simulink library "lib_discrete_time_PI_controller"  (R2023a)
settings: Solver=VariableStepAuto  StartTime=0.0  StopTime=10.0  RelTol=1e-3
undefined symbols (not defined in the file): bit
libraries: lib_conversion x11, lib_dynamic_saturator x4, lib_discrete_time_integrator x4
settings Model: Creator=cav2ofo  LastModifiedBy=xiaoqiang.yuan
settings OptimizationCC: ReuseModelBlockBuffer=off

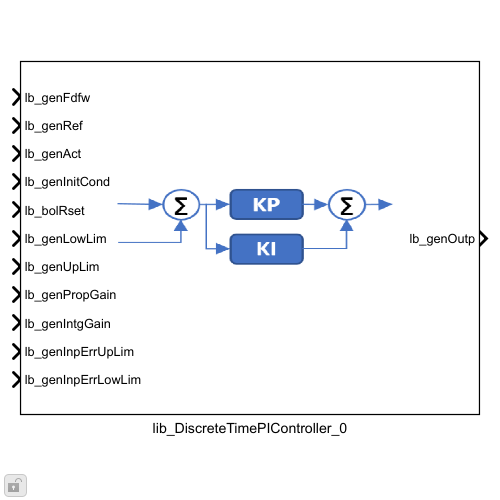
[thumbnail: Simulink's stored preview of the top-level diagram]
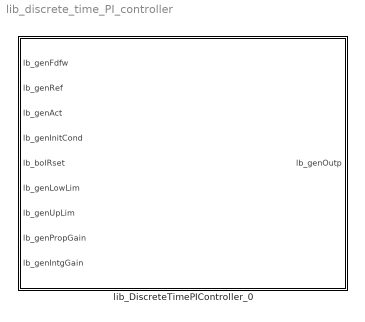
== system lib_discrete_time_PI_controller ==
  lib_DiscreteTimePIController_0 : Subsystem  mask{lb_parSampTime=0.01, lb_parMaxSampTime=0.1, lb_parMaxPropGain=1, lb_parMaxIntgGain=1, lb_parRefInpMaxVal=1000, lb_parRefInpMinVal=-1000, lb_parMaxErrVal=2*1000, lb_parMinErrVal=-2*1000, lb_parMaxOutpVal=20, lb_parMinOutpVal=-20, lb_parAccmDataTypeMode=32-bit, lb_parOutpDataType=fixdt(1,16,2^0,0), lb_parSatMode=anti-windup with back-calculation}
      mask prompts: lb_parSampTime "Sampling time [s]:"; lb_parMaxSampTime "Maximum sampling time [s]:"; lb_parMaxPropGain "Maximum proportional gain (kp):"; lb_parMaxIntgGain "Maximum integral gain [ou/(iu*s)]:"; lb_parRefInpMaxVal "Reference input maximum value [iu]:"; lb_parRefInpMinVal "Reference input minimum value [iu]:"; lb_parMaxErrVal "Maximum error (Ref-Act) value [iu]:"; lb_parMinErrVal "Minimum error (Ref-Act) value [iu]:"; lb_parMaxOutpVal "Maximum output value [ou]:"; lb_parMinOutpVal "Minimum output value [ou]:"; lb_parAccmDataTypeMode "Accumulator data type mode:"; lb_parOutpDataType "Output data type:"; lb_parSatMode "Output saturation mode:"
      mask init:
      | % =======================================================
      | % This script is a script to flags output saturation
      | % when either the output saturation without anti-windup
      | % or custom anti-windup method is selected. It also computes
      | % custom datatypes required for intermediate calcuations
      | % Author: Niraj Rathod
      | % Date: 19/07/2022
      | % =======================================================
      | % Enable saturation flag in case of saturation 
      | % without anti-windup (2) or custom anti-windup method (4)
      | % if lb_parAntiWdpMtd == 2 ||  lb_parAntiWdpMtd == 4
      | %    set_param(gcb,'lb_parSatFlag', 'on');
      | % else
      | %    set_param(gcb,'lb_parSatFlag', 'off');
      | % end
      | 
      | % Setting the maximum sampling time equal to the user define sampling time
      | % value
      | lb_parMaxSampTime = double(lb_parSampTime);
      | 
      | % Data type slope for the diffference between unstaurated 
      | % and saturated output signal used by anti-windup 
      | % with back-calculation
      | lb_outpDiffDataType = Simulink.NumericType;
      | lb_outpDiffDataType.DataTypeMode = 'Fixed-point: slope and bias scaling';
      | lb_outpDiffDataType.Slope = lb_parOutpDataType.Slope*2; 
      | 
      | % Min/max value for accumulator datatype
      | lb_parAccmMaxOutp = 3*double(lb_parRefInpMaxVal);
      | lb_parAccmMinOutp = 3*double(lb_parRefInpMinVal);
      | 
      | 
      | %% Activate variant subsystem choice by means of set_param function
      | % switch lb_parSatMode
      | %     
      | %     case 'none' 
      | %         
      | %         set_param([gcb,'/vss_PIControllerModes'],'VariantControl', 'VSS_MODE == 1')
      | %         set_param(gcb,'lb_parSatFlag', 'off');
      | % 
      | %     case 'output saturation without anti-windup'
      | % 
      | %         set_param([gcb,'/vss_PIControllerModes'],'VariantControl', 'VSS_MODE == 1')
      | %         set_param(gcb,'lb_parSatFlag', 'on');
      | % 
      | %     case 'anti-windup with custom algorithm'
      | %         
      | %         set_param([gcb,'/vss_PIControllerModes'],'VariantControl', 'VSS_MODE == 2')
      | %         set_param(gcb,'lb_parSatFlag', 'off');
      | %         
      | %     case 'Integral control'
      | %         
      | %         set_param([gcb,'/vss_PIControllerModes'],'VariantControl', 'VSS_MODE == 3')
      | %         set_param(gcb,'lb_parSatFlag', 'off');
      | %         
      | % end
      mask TypeOptions lb_parMaxSampTime: vss_PIControllerModes/vss_NoSaturation/lib_DiscreteTimeIntegrator_1/lb_parMaxSampTime | vss_PIControllerModes/vss_SaturationBackCalcAntiWindup/lib_DiscreteTimeIntegrator_1/lb_parMaxSampTime | vss_PIControllerModes/vss_SaturationCustomAntiWindup/lib_DiscreteTimeIntegrator_1/lb_parMaxSampTime | vss_PIControllerModes/vss_SaturationNoAntiWindup/lib_DiscreteTimeIntegrator_1/lb_parMaxSampTime
      mask TypeOptions lb_parMaxIntgGain: vss_PIControllerModes/vss_NoSaturation/lib_DiscreteTimeIntegrator_1/lb_parMaxIntgGain | vss_PIControllerModes/vss_SaturationBackCalcAntiWindup/lib_DiscreteTimeIntegrator_1/lb_parMaxIntgGain | vss_PIControllerModes/vss_SaturationCustomAntiWindup/lib_DiscreteTimeIntegrator_1/lb_parMaxIntgGain | vss_PIControllerModes/vss_SaturationNoAntiWindup/lib_DiscreteTimeIntegrator_1/lb_parMaxIntgGain
      mask TypeOptions lb_parAccmDataTypeMode: vss_PIControllerModes/vss_NoSaturation/lib_DiscreteTimeIntegrator_1/lb_parAccmDataTypeMode | vss_PIControllerModes/vss_SaturationBackCalcAntiWindup/lib_DiscreteTimeIntegrator_1/lb_parAccmDataTypeMode | vss_PIControllerModes/vss_SaturationCustomAntiWindup/lib_DiscreteTimeIntegrator_1/lb_parAccmDataTypeMode | vss_PIControllerModes/vss_SaturationNoAntiWindup/lib_DiscreteTimeIntegrator_1/lb_parAccmDataTypeMode
      mask TypeOptions lb_parSatMode: none | output saturation without anti-windup | anti-windup with back-calculation | anti-windup with custom algorithm
      mask DialogControl DescGroupVar Prompt: Proportional-Integral (PI) Controller
      mask DialogControl DescTextVar Prompt: VHIT Control Library
      mask DialogControl piDesc Prompt: This is a Custom Proportional-Integral (PI) block developed for the motor control.
      mask DialogControl blockParam Prompt: Parameters
      mask DialogControl dataTypeDesc Prompt: Data type
      mask DialogControl oprModDesc Prompt: Operating modes
      mask Display: image('PiController.png')

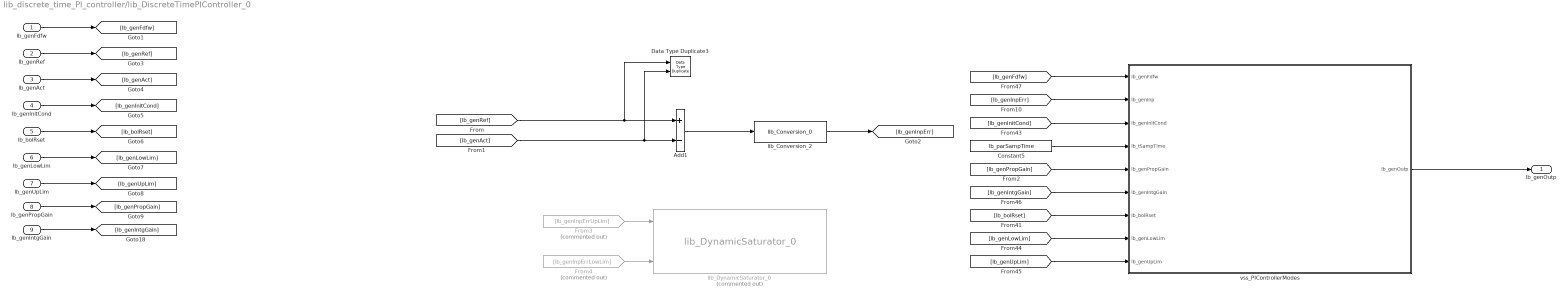
== system lib_discrete_time_PI_controller/lib_DiscreteTimePIController_0 ==
  lb_genFdfw : Inport  OutDataTypeStr=lb_parOutpDataType
  lb_genRef : Inport  Port=2  OutMin=lb_parRefInpMinVal  OutMax=lb_parRefInpMaxVal
  lb_genAct : Inport  Port=3  OutMin=lb_parRefInpMinVal  OutMax=lb_parRefInpMaxVal
  lb_genInitCond : Inport  Port=4  OutDataTypeStr=lb_parOutpDataType
  lb_bolRset : Inport  Port=5  OutDataTypeStr=boolean
  lb_genLowLim : Inport  Port=6  OutDataTypeStr=lb_parOutpDataType
  lb_genUpLim : Inport  Port=7  OutDataTypeStr=lb_parOutpDataType
  lb_genPropGain : Inport  Port=8  OutMin=0  OutMax=lb_parMaxPropGain
  lb_genIntgGain : Inport  Port=9  OutMin=0  OutMax=lb_parMaxIntgGain
  Add1 : Sum  Inputs=+-  OutDataTypeStr=Inherit: Inherit via back propagation  RndMeth=Simplest
  Constant5 : Constant  Value=lb_parSampTime
  Data Type Duplicate3 : DataTypeDuplicate
  From3 : From  Commented=on  GotoTag=lb_genInpErrUpLim
  From4 : From  Commented=on  GotoTag=lb_genInpErrLowLim
  lib_Conversion_2 : lib_conversion/lib_Conversion_0  lb_parDataType=fixdt(1,16)  lb_parOutpMaxVal=2*lb_parRefInpMaxVal  lb_parOutpMinVal=2*lb_parRefInpMinVal  lb_parSatFlag=off
  lib_DynamicSaturator_0 : lib_dynamic_saturator/lib_DynamicSaturator_0  Commented=on
  vss_PIControllerModes : Subsystem  Variant=on
  lb_genOutp : Outport  VectorParamsAs1DForOutWhenUnconnected=off
  wires:
  [lb_genPropGain] -> vss_PIControllerModes/5(lb_genPropGain)
  lb_genPropGain/1 -> [lb_genPropGain]
  lb_genLowLim/1 -> [lb_genLowLim]
  lb_genUpLim/1 -> [lb_genUpLim]
  [lb_genAct] -> Data Type Duplicate3/2, Add1/2
  [lb_genRef] -> Add1/1, Data Type Duplicate3/1
  lb_genRef/1 -> [lb_genRef]
  lb_genAct/1 -> [lb_genAct]
  lb_genInitCond/1 -> [lb_genInitCond]
  lb_bolRset/1 -> [lb_bolRset]
  lb_genFdfw/1 -> [lb_genFdfw]
  lb_genIntgGain/1 -> [lb_genIntgGain]
  [lb_genInpErr] -> vss_PIControllerModes/2(lb_genInp)
  [lb_genInitCond] -> vss_PIControllerModes/3(lb_genInitCond)
  Constant5/1 -> vss_PIControllerModes/4(lb_tSampTime)
  [lb_genIntgGain] -> vss_PIControllerModes/6(lb_genIntgGain)
  [lb_bolRset] -> vss_PIControllerModes/7(lb_bolRset)
  [lb_genLowLim] -> vss_PIControllerModes/8(lb_genLowLim)
  [lb_genUpLim] -> vss_PIControllerModes/9(lb_genUpLim)
  [lb_genFdfw] -> vss_PIControllerModes/1(lb_genFdfw)
  vss_PIControllerModes/1(lb_genOutp) -> lb_genOutp/1
  From3/1 -> lib_DynamicSaturator_0/1
  From4/1 -> lib_DynamicSaturator_0/3
  lib_Conversion_2/1 -> [lb_genInpErr]
  Add1/1 -> lib_Conversion_2/1

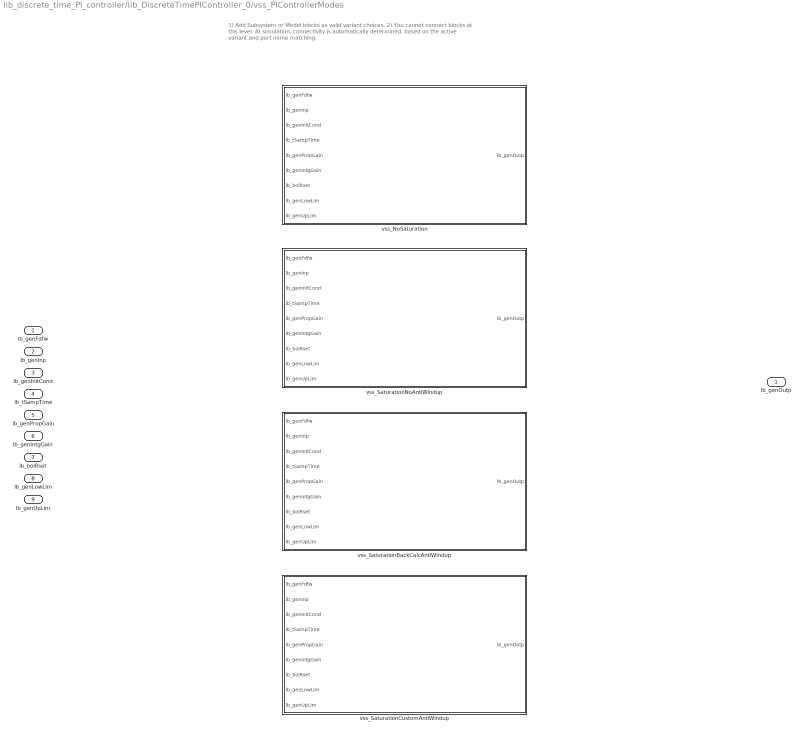
== system lib_discrete_time_PI_controller/lib_DiscreteTimePIController_0/vss_PIControllerModes ==
  note: 1) Add Subsystem or Model blocks as valid variant choices.
      | 2) You cannot connect blocks at this level. At simulation, connectivity is automatically
      | determined, based on the active variant and port name matching.
  lb_genFdfw : Inport
  lb_genInp : Inport  Port=2
  lb_genInitCond : Inport  Port=3
  lb_tSampTime : Inport  Port=4
  lb_genPropGain : Inport  Port=5
  lb_genIntgGain : Inport  Port=6
  lb_bolRset : Inport  Port=7
  lb_genLowLim : Inport  Port=8
  lb_genUpLim : Inport  Port=9
  vss_NoSaturation : Subsystem  VariantControl=lb_parSatMode == 1
  vss_SaturationBackCalcAntiWindup : Subsystem  VariantControl=lb_parSatMode == 3
  vss_SaturationCustomAntiWindup : Subsystem  VariantControl=lb_parSatMode == 4
  vss_SaturationNoAntiWindup : Subsystem  VariantControl=lb_parSatMode == 2
  lb_genOutp : Outport

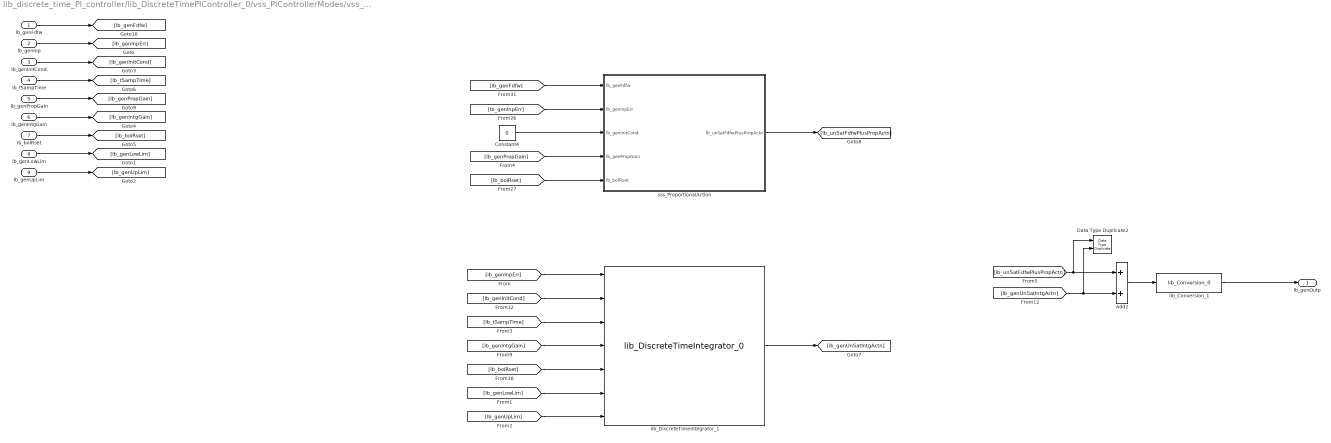
== system lib_discrete_time_PI_controller/lib_DiscreteTimePIController_0/vss_PIControllerModes/vss_NoSaturation ==
  lb_genFdfw : Inport
  lb_genInp : Inport  Port=2
  lb_genInitCond : Inport  Port=3
  lb_tSampTime : Inport  Port=4
  lb_genPropGain : Inport  Port=5
  lb_genIntgGain : Inport  Port=6
  lb_bolRset : Inport  Port=7
  lb_genLowLim : Inport  Port=8
  lb_genUpLim : Inport  Port=9
  Add2 : Sum  OutDataTypeStr=Inherit: Inherit via back propagation  RndMeth=Simplest
  Constant4 : Constant  Value=0  OutDataTypeStr=lb_parOutpDataType
  Data Type Duplicate2 : DataTypeDuplicate
  lib_Conversion_1 : lib_conversion/lib_Conversion_0  lb_parDataType=lb_parOutpDataType  lb_parOutpMaxVal=[]  lb_parOutpMinVal=[]  lb_parSatFlag=off
  lib_DiscreteTimeIntegrator_1 : lib_discrete_time_integrator/lib_DiscreteTimeIntegrator_0  lb_parMaxInpVal=lb_parMaxErrVal  lb_parMinInpVal=lb_parMinErrVal  lb_parMaxSampTime=lb_parMaxSampTime  lb_parMaxIntgGain=lb_parMaxIntgGain  lb_parAccmDataTypeMode=32-bit  lb_parOutpDataType=lb_parOutpDataType  lb_parIntgScopMode=Integral control  lb_parSatFlag=off
      settings: LibrarySourceBlock=vhit_control_library/lib_DiscreteTimeIntegrator_0
  sss_ProportionalAction : Subsystem
  lb_genOutp : Outport  VectorParamsAs1DForOutWhenUnconnected=off
  wires:
  [lb_genPropGain] -> sss_ProportionalAction/4(lb_genPropGain)
  lb_genPropGain/1 -> [lb_genPropGain]
  [lb_bolRset] -> lib_DiscreteTimeIntegrator_1/5
  [lb_genInpErr] -> lib_DiscreteTimeIntegrator_1/1
  [lb_genLowLim] -> lib_DiscreteTimeIntegrator_1/6
  [lb_genInitCond] -> lib_DiscreteTimeIntegrator_1/2
  [lb_genIntgGain] -> lib_DiscreteTimeIntegrator_1/4
  [lb_tSampTime] -> lib_DiscreteTimeIntegrator_1/3
  lib_DiscreteTimeIntegrator_1/1 -> [lb_genUnSatIntgActn]
  [lb_genUpLim] -> lib_DiscreteTimeIntegrator_1/7
  [lb_genInpErr] -> sss_ProportionalAction/2(lb_genInpErr)
  [lb_bolRset] -> sss_ProportionalAction/5(lb_bolRset)
  [lb_genFdfw] -> sss_ProportionalAction/1(lb_genFdfw)
  sss_ProportionalAction/1(lb_unSatFdfwPlusPropActn) -> [lb_unSatFdfwPlusPropActn]
  Constant4/1 -> sss_ProportionalAction/3(lb_genInitCond)
  Add2/1 -> lib_Conversion_1/1
  [lb_unSatFdfwPlusPropActn] -> Data Type Duplicate2/1, Add2/1
  [lb_genUnSatIntgActn] -> Add2/2, Data Type Duplicate2/2
  lib_Conversion_1/1 -> lb_genOutp/1
  lb_genInp/1 -> [lb_genInpErr]
  lb_genInitCond/1 -> [lb_genInitCond]
  lb_tSampTime/1 -> [lb_tSampTime]
  lb_genIntgGain/1 -> [lb_genIntgGain]
  lb_bolRset/1 -> [lb_bolRset]
  lb_genLowLim/1 -> [lb_genLowLim]
  lb_genUpLim/1 -> [lb_genUpLim]
  lb_genFdfw/1 -> [lb_genFdfw]

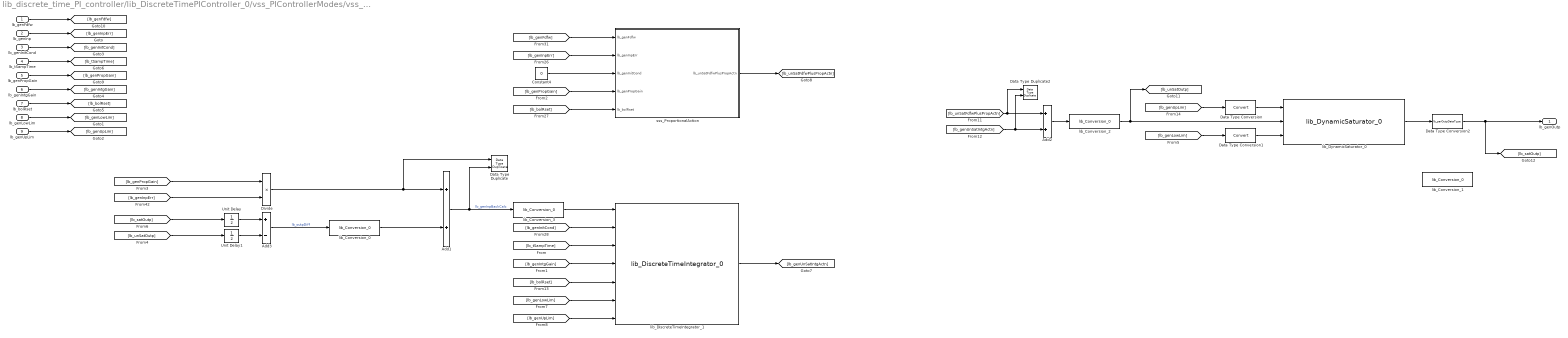
== system lib_discrete_time_PI_controller/lib_DiscreteTimePIController_0/vss_PIControllerModes/vss_SaturationBackCalcAntiWindup ==
  lb_genFdfw : Inport
  lb_genInp : Inport  Port=2
  lb_genInitCond : Inport  Port=3
  lb_tSampTime : Inport  Port=4
  lb_genPropGain : Inport  Port=5
  lb_genIntgGain : Inport  Port=6
  lb_bolRset : Inport  Port=7
  lb_genLowLim : Inport  Port=8
  lb_genUpLim : Inport  Port=9
  Add1 : Sum  OutDataTypeStr=Inherit: Inherit via back propagation  RndMeth=Simplest
  Add2 : Sum  OutDataTypeStr=Inherit: Inherit via back propagation  RndMeth=Simplest
  Add3 : Sum  Inputs=+-  OutDataTypeStr=Inherit: Inherit via back propagation  RndMeth=Simplest
  Constant4 : Constant  Value=0  OutDataTypeStr=Inherit: Inherit via back propagation
  Data Type Duplicate : DataTypeDuplicate
  Data Type Duplicate2 : DataTypeDuplicate
  Data Type Conversion : DataTypeConversion  SaturateOnIntegerOverflow=off  RndMeth=Floor
  Data Type Conversion1 : DataTypeConversion  SaturateOnIntegerOverflow=off  RndMeth=Floor
  Data Type Conversion2 : DataTypeConversion  OutDataTypeStr=lb_parOutpDataType  SaturateOnIntegerOverflow=off  RndMeth=Floor
  Divide : Product  Inputs=**  OutDataTypeStr=Inherit: Inherit via back propagation
  Unit Delay : UnitDelay  SampleTime=-1  HasFrameUpgradeWarning=on
  Unit Delay1 : UnitDelay  SampleTime=-1  HasFrameUpgradeWarning=on
  lib_Conversion_0 : lib_conversion/lib_Conversion_0  lb_parDataType=lb_outpDiffDataType  lb_parOutpMaxVal=[]  lb_parOutpMinVal=[]  lb_parSatFlag=off
  lib_Conversion_1 : lib_conversion/lib_Conversion_0  lb_parDataType=lb_parOutpDataType  lb_parOutpMaxVal=[]  lb_parOutpMinVal=[]  lb_parSatFlag=off
  lib_Conversion_2 : lib_conversion/lib_Conversion_0  lb_parDataType=lb_outpDiffDataType  lb_parOutpMaxVal=[]  lb_parOutpMinVal=[]  lb_parSatFlag=off
  lib_Conversion_3 : lib_conversion/lib_Conversion_0  lb_parDataType=lb_parOutpDataType  lb_parOutpMaxVal=[]  lb_parOutpMinVal=[]  lb_parSatFlag=off
  lib_DiscreteTimeIntegrator_1 : lib_discrete_time_integrator/lib_DiscreteTimeIntegrator_0  lb_parMaxInpVal=lb_parMaxOutpVal  lb_parMinInpVal=-lb_parMaxOutpVal  lb_parMaxSampTime=lb_parMaxSampTime  lb_parMaxIntgGain=lb_parMaxIntgGain  lb_parAccmDataTypeMode=32-bit  lb_parOutpDataType=lb_parOutpDataType  lb_parIntgScopMode=Integral control  lb_parSatFlag=off
      settings: LibrarySourceBlock=vhit_control_library/lib_DiscreteTimeIntegrator_0
  lib_DynamicSaturator_0 : lib_dynamic_saturator/lib_DynamicSaturator_0
  sss_ProportionalAction : Subsystem
  lb_genOutp : Outport  VectorParamsAs1DForOutWhenUnconnected=off
  wires:
  [lb_genInpErr] -> sss_ProportionalAction/2(lb_genInpErr)
  Constant4/1 -> sss_ProportionalAction/3(lb_genInitCond)
  sss_ProportionalAction/1(lb_unSatFdfwPlusPropActn) -> [lb_unSatFdfwPlusPropActn]
  [lb_bolRset] -> sss_ProportionalAction/5(lb_bolRset)
  [lb_genFdfw] -> sss_ProportionalAction/1(lb_genFdfw)
  [lb_genPropGain] -> sss_ProportionalAction/4(lb_genPropGain)
  lb_genPropGain/1 -> [lb_genPropGain]
  lb_genIntgGain/1 -> [lb_genIntgGain]
  Data Type Conversion2/1 -> lb_genOutp/1, [lb_satOutp]
  lb_genFdfw/1 -> [lb_genFdfw]
  lb_genUpLim/1 -> [lb_genUpLim]
  lb_genInitCond/1 -> [lb_genInitCond]
  lb_bolRset/1 -> [lb_bolRset]
  lb_genInp/1 -> [lb_genInpErr]
  lb_genLowLim/1 -> [lb_genLowLim]
  lb_tSampTime/1 -> [lb_tSampTime]
  lib_DiscreteTimeIntegrator_1/1 -> [lb_genUnSatIntgActn]
  [lb_tSampTime] -> lib_DiscreteTimeIntegrator_1/3
  [lb_unSatOutp] -> Unit Delay1/1
  Add3/1 -> lib_Conversion_0/1  "lb_outpDiff"
  Add1/1 -> lib_Conversion_3/1, Data Type Duplicate/2  "lb_genInpBackCalc"
  Divide/1 -> Add1/1, Data Type Duplicate/1
  [lb_satOutp] -> Unit Delay/1
  [lb_bolRset] -> lib_DiscreteTimeIntegrator_1/5
  lib_Conversion_3/1 -> lib_DiscreteTimeIntegrator_1/1
  [lb_genInpErr] -> Divide/2
  [lb_genIntgGain] -> lib_DiscreteTimeIntegrator_1/4
  [lb_genInitCond] -> lib_DiscreteTimeIntegrator_1/2
  [lb_genUnSatIntgActn] -> Add2/2, Data Type Duplicate2/2
  lib_DynamicSaturator_0/1 -> Data Type Conversion2/1
  [lb_genLowLim] -> Data Type Conversion1/1
  [lb_genUpLim] -> Data Type Conversion/1
  [lb_unSatFdfwPlusPropActn] -> Data Type Duplicate2/1, Add2/1
  [lb_genLowLim] -> lib_DiscreteTimeIntegrator_1/6
  [lb_genUpLim] -> lib_DiscreteTimeIntegrator_1/7
  Unit Delay/1 -> Add3/1
  Unit Delay1/1 -> Add3/2
  [lb_genPropGain] -> Divide/1
  lib_Conversion_0/1 -> Add1/2
  Add2/1 -> lib_Conversion_2/1
  lib_Conversion_2/1 -> [lb_unSatOutp], lib_DynamicSaturator_0/2
  Data Type Conversion/1 -> lib_DynamicSaturator_0/1
  Data Type Conversion1/1 -> lib_DynamicSaturator_0/3

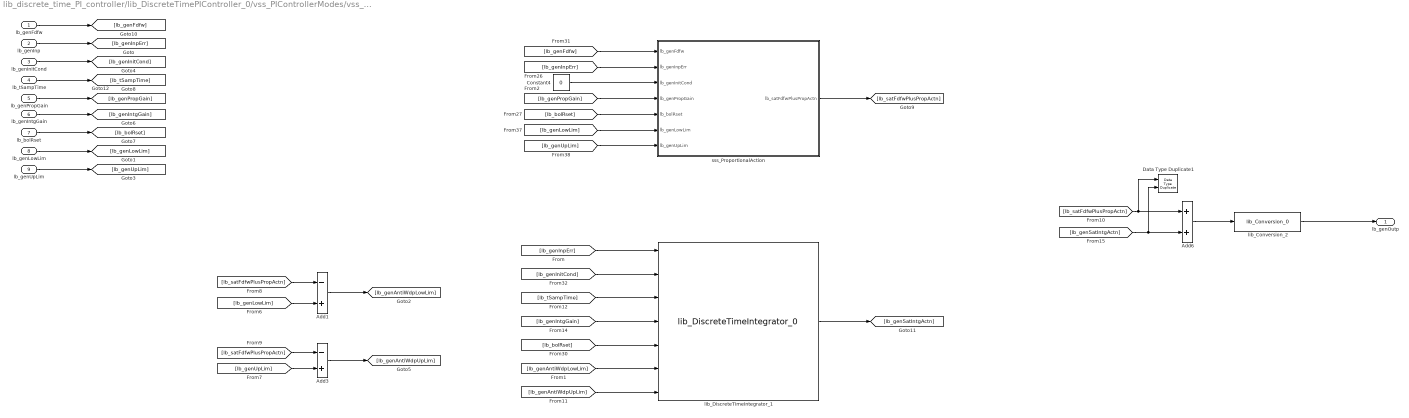
== system lib_discrete_time_PI_controller/lib_DiscreteTimePIController_0/vss_PIControllerModes/vss_SaturationCustomAntiWindup ==
  lb_genFdfw : Inport
  lb_genInp : Inport  Port=2
  lb_genInitCond : Inport  Port=3
  lb_tSampTime : Inport  Port=4
  lb_genPropGain : Inport  Port=5
  lb_genIntgGain : Inport  Port=6
  lb_bolRset : Inport  Port=7
  lb_genLowLim : Inport  Port=8
  lb_genUpLim : Inport  Port=9
  Add1 : Sum  Inputs=-+  OutDataTypeStr=Inherit: Inherit via back propagation  RndMeth=Simplest  SaturateOnIntegerOverflow=on
  Add3 : Sum  Inputs=-+  OutDataTypeStr=Inherit: Inherit via back propagation  RndMeth=Simplest  SaturateOnIntegerOverflow=on
  Add6 : Sum  OutDataTypeStr=Inherit: Inherit via back propagation  RndMeth=Simplest
  Constant4 : Constant  Value=0  OutDataTypeStr=lb_parOutpDataType
  Data Type Duplicate1 : DataTypeDuplicate
  lib_Conversion_2 : lib_conversion/lib_Conversion_0  lb_parDataType=lb_parOutpDataType  lb_parOutpMaxVal=[]  lb_parOutpMinVal=[]  lb_parSatFlag=off
  lib_DiscreteTimeIntegrator_1 : lib_discrete_time_integrator/lib_DiscreteTimeIntegrator_0  lb_parMaxInpVal=lb_parMaxErrVal  lb_parMinInpVal=lb_parMinErrVal  lb_parMaxSampTime=lb_parMaxSampTime  lb_parMaxIntgGain=lb_parMaxIntgGain  lb_parAccmDataTypeMode=32-bit  lb_parOutpDataType=lb_parOutpDataType  lb_parIntgScopMode=Integral control  lb_parSatFlag=on
      settings: LibrarySourceBlock=vhit_control_library/lib_DiscreteTimeIntegrator_0
  sss_ProportionalAction : Subsystem
  lb_genOutp : Outport  VectorParamsAs1DForOutWhenUnconnected=off
  wires:
  sss_ProportionalAction/1(lb_satFdfwPlusPropActn) -> [lb_satFdfwPlusPropActn]
  [lb_genUpLim] -> sss_ProportionalAction/7(lb_genUpLim)
  [lb_genInpErr] -> sss_ProportionalAction/2(lb_genInpErr)
  [lb_bolRset] -> sss_ProportionalAction/5(lb_bolRset)
  [lb_genFdfw] -> sss_ProportionalAction/1(lb_genFdfw)
  Constant4/1 -> sss_ProportionalAction/3(lb_genInitCond)
  [lb_genLowLim] -> sss_ProportionalAction/6(lb_genLowLim)
  [lb_genPropGain] -> sss_ProportionalAction/4(lb_genPropGain)
  lb_genPropGain/1 -> [lb_genPropGain]
  lb_tSampTime/1 -> [lb_tSampTime]
  lb_genLowLim/1 -> [lb_genLowLim]
  lb_bolRset/1 -> [lb_bolRset]
  lb_genUpLim/1 -> [lb_genUpLim]
  lib_Conversion_2/1 -> lb_genOutp/1
  lb_genIntgGain/1 -> [lb_genIntgGain]
  lb_genFdfw/1 -> [lb_genFdfw]
  lb_genInp/1 -> [lb_genInpErr]
  lb_genInitCond/1 -> [lb_genInitCond]
  [lb_genLowLim] -> Add1/2
  [lb_genUpLim] -> Add3/2
  Add1/1 -> [lb_genAntiWdpLowLim]
  [lb_satFdfwPlusPropActn] -> Add1/1
  [lb_satFdfwPlusPropActn] -> Add3/1
  Add3/1 -> [lb_genAntiWdpUpLim]
  [lb_satFdfwPlusPropActn] -> Data Type Duplicate1/1, Add6/1
  [lb_genSatIntgActn] -> Add6/2, Data Type Duplicate1/2
  Add6/1 -> lib_Conversion_2/1
  [lb_genInitCond] -> lib_DiscreteTimeIntegrator_1/2
  [lb_bolRset] -> lib_DiscreteTimeIntegrator_1/5
  [lb_genIntgGain] -> lib_DiscreteTimeIntegrator_1/4
  [lb_genAntiWdpUpLim] -> lib_DiscreteTimeIntegrator_1/7
  [lb_genInpErr] -> lib_DiscreteTimeIntegrator_1/1
  [lb_tSampTime] -> lib_DiscreteTimeIntegrator_1/3
  [lb_genAntiWdpLowLim] -> lib_DiscreteTimeIntegrator_1/6
  lib_DiscreteTimeIntegrator_1/1 -> [lb_genSatIntgActn]

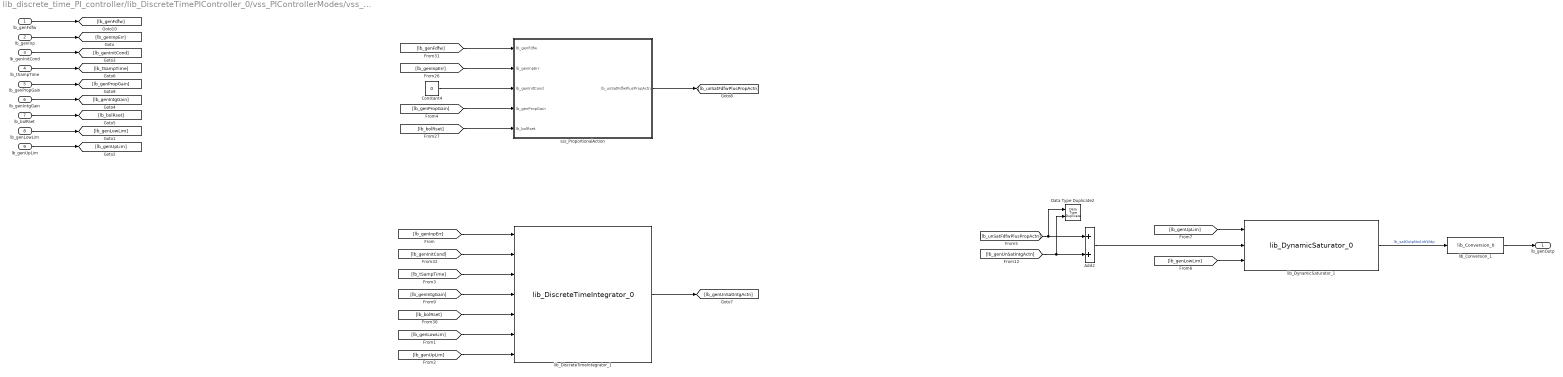
== system lib_discrete_time_PI_controller/lib_DiscreteTimePIController_0/vss_PIControllerModes/vss_SaturationNoAntiWindup ==
  lb_genFdfw : Inport
  lb_genInp : Inport  Port=2
  lb_genInitCond : Inport  Port=3
  lb_tSampTime : Inport  Port=4
  lb_genPropGain : Inport  Port=5
  lb_genIntgGain : Inport  Port=6
  lb_bolRset : Inport  Port=7
  lb_genLowLim : Inport  Port=8
  lb_genUpLim : Inport  Port=9
  Add2 : Sum  OutDataTypeStr=Inherit: Inherit via back propagation  RndMeth=Simplest
  Constant4 : Constant  Value=0  OutDataTypeStr=lb_parOutpDataType
  Data Type Duplicate2 : DataTypeDuplicate
  lib_Conversion_1 : lib_conversion/lib_Conversion_0  lb_parDataType=lb_parOutpDataType  lb_parOutpMaxVal=[]  lb_parOutpMinVal=[]  lb_parSatFlag=off
  lib_DiscreteTimeIntegrator_1 : lib_discrete_time_integrator/lib_DiscreteTimeIntegrator_0  lb_parMaxInpVal=lb_parMaxErrVal  lb_parMinInpVal=lb_parMinErrVal  lb_parMaxSampTime=lb_parMaxSampTime  lb_parMaxIntgGain=lb_parMaxIntgGain  lb_parAccmDataTypeMode=32-bit  lb_parOutpDataType=lb_parOutpDataType  lb_parIntgScopMode=Integral control  lb_parSatFlag=off
      settings: LibrarySourceBlock=vhit_control_library/lib_DiscreteTimeIntegrator_0
  lib_DynamicSaturator_1 : lib_dynamic_saturator/lib_DynamicSaturator_0
  sss_ProportionalAction : Subsystem
  lb_genOutp : Outport  VectorParamsAs1DForOutWhenUnconnected=off
  wires:
  [lb_genInpErr] -> sss_ProportionalAction/2(lb_genInpErr)
  Constant4/1 -> sss_ProportionalAction/3(lb_genInitCond)
  sss_ProportionalAction/1(lb_unSatFdfwPlusPropActn) -> [lb_unSatFdfwPlusPropActn]
  [lb_bolRset] -> sss_ProportionalAction/5(lb_bolRset)
  [lb_genFdfw] -> sss_ProportionalAction/1(lb_genFdfw)
  [lb_genPropGain] -> sss_ProportionalAction/4(lb_genPropGain)
  lb_genPropGain/1 -> [lb_genPropGain]
  [lb_bolRset] -> lib_DiscreteTimeIntegrator_1/5
  [lb_genInpErr] -> lib_DiscreteTimeIntegrator_1/1
  [lb_genLowLim] -> lib_DiscreteTimeIntegrator_1/6
  [lb_genInitCond] -> lib_DiscreteTimeIntegrator_1/2
  [lb_genIntgGain] -> lib_DiscreteTimeIntegrator_1/4
  [lb_tSampTime] -> lib_DiscreteTimeIntegrator_1/3
  lib_DiscreteTimeIntegrator_1/1 -> [lb_genUnSatIntgActn]
  [lb_genUpLim] -> lib_DiscreteTimeIntegrator_1/7
  Add2/1 -> lib_DynamicSaturator_1/2
  [lb_genLowLim] -> lib_DynamicSaturator_1/3
  [lb_unSatFdfwPlusPropActn] -> Data Type Duplicate2/1, Add2/1
  [lb_genUnSatIntgActn] -> Add2/2, Data Type Duplicate2/2
  [lb_genUpLim] -> lib_DynamicSaturator_1/1
  lib_Conversion_1/1 -> lb_genOutp/1
  lb_genInp/1 -> [lb_genInpErr]
  lb_genInitCond/1 -> [lb_genInitCond]
  lb_tSampTime/1 -> [lb_tSampTime]
  lb_genIntgGain/1 -> [lb_genIntgGain]
  lb_bolRset/1 -> [lb_bolRset]
  lb_genLowLim/1 -> [lb_genLowLim]
  lb_genUpLim/1 -> [lb_genUpLim]
  lb_genFdfw/1 -> [lb_genFdfw]
  lib_DynamicSaturator_1/1 -> lib_Conversion_1/1  "lb_satOutpNoAntiWdp"

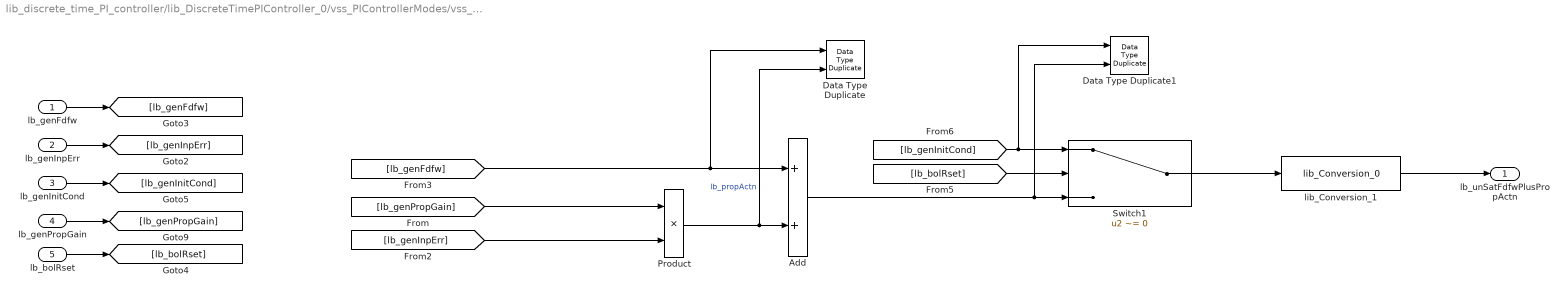
== system lib_discrete_time_PI_controller/lib_DiscreteTimePIController_0/vss_PIControllerModes/vss_NoSaturation/sss_ProportionalAction ==
  lb_genFdfw : Inport
  lb_genInpErr : Inport  Port=2
  lb_genInitCond : Inport  Port=3
  lb_genPropGain : Inport  Port=4
  lb_bolRset : Inport  Port=5
  Add : Sum  RndMeth=Simplest  OutDataTypeStr=Inherit: Same as first input
  Data Type Duplicate : DataTypeDuplicate
  Data Type Duplicate1 : DataTypeDuplicate
  Product : Product  OutDataTypeStr=Inherit: Inherit via back propagation  RndMeth=Simplest
  Switch1 : Switch  Criteria=u2 ~= 0  OutDataTypeStr=Inherit: Inherit via back propagation  SaturateOnIntegerOverflow=off  InputSameDT=off
  lib_Conversion_1 : lib_conversion/lib_Conversion_0  lb_parDataType=lb_parOutpDataType  lb_parOutpMaxVal=[]  lb_parOutpMinVal=[]  lb_parSatFlag=off
  lb_unSatFdfwPlusPropActn : Outport
  wires:
  [lb_genPropGain] -> Product/1
  lb_genPropGain/1 -> [lb_genPropGain]
  lib_Conversion_1/1 -> lb_unSatFdfwPlusPropActn/1
  lb_bolRset/1 -> [lb_bolRset]
  Switch1/1 -> lib_Conversion_1/1
  [lb_genInitCond] -> Switch1/1, Data Type Duplicate1/1
  [lb_bolRset] -> Switch1/2
  lb_genInpErr/1 -> [lb_genInpErr]
  lb_genFdfw/1 -> [lb_genFdfw]
  Product/1 -> Data Type Duplicate/2, Add/2  "lb_propActn"
  [lb_genFdfw] -> Data Type Duplicate/1, Add/1
  [lb_genInpErr] -> Product/2
  Add/1 -> Switch1/3, Data Type Duplicate1/2
  lb_genInitCond/1 -> [lb_genInitCond]

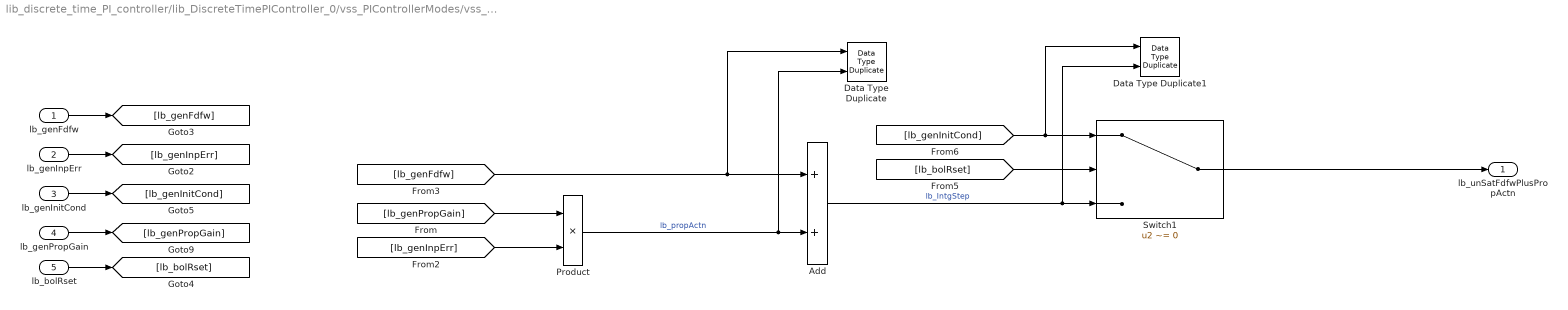
== system lib_discrete_time_PI_controller/lib_DiscreteTimePIController_0/vss_PIControllerModes/vss_SaturationBackCalcAntiWindup/sss_ProportionalAction ==
  lb_genFdfw : Inport
  lb_genInpErr : Inport  Port=2
  lb_genInitCond : Inport  Port=3
  lb_genPropGain : Inport  Port=4
  lb_bolRset : Inport  Port=5
  Add : Sum  RndMeth=Simplest  OutDataTypeStr=Inherit: Same as first input
  Data Type Duplicate : DataTypeDuplicate
  Data Type Duplicate1 : DataTypeDuplicate
  Product : Product  OutDataTypeStr=Inherit: Inherit via back propagation  RndMeth=Simplest
  Switch1 : Switch  Criteria=u2 ~= 0  OutDataTypeStr=Inherit: Inherit via back propagation  SaturateOnIntegerOverflow=off  InputSameDT=off
  lb_unSatFdfwPlusPropActn : Outport
  wires:
  lb_genInitCond/1 -> [lb_genInitCond]
  [lb_genInpErr] -> Product/2
  Product/1 -> Add/2, Data Type Duplicate/2  "lb_propActn"
  lb_genFdfw/1 -> [lb_genFdfw]
  lb_genInpErr/1 -> [lb_genInpErr]
  [lb_bolRset] -> Switch1/2
  [lb_genInitCond] -> Data Type Duplicate1/1, Switch1/1
  lb_bolRset/1 -> [lb_bolRset]
  Switch1/1 -> lb_unSatFdfwPlusPropActn/1
  lb_genPropGain/1 -> [lb_genPropGain]
  [lb_genPropGain] -> Product/1
  Add/1 -> Data Type Duplicate1/2, Switch1/3  "lb_IntgStep"
  [lb_genFdfw] -> Add/1, Data Type Duplicate/1

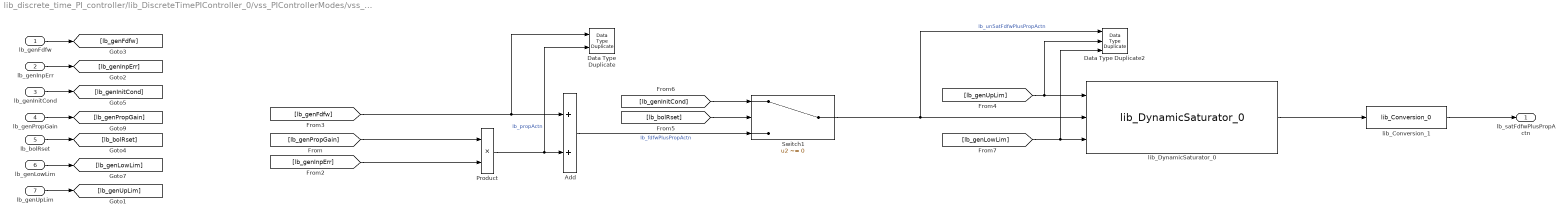
== system lib_discrete_time_PI_controller/lib_DiscreteTimePIController_0/vss_PIControllerModes/vss_SaturationCustomAntiWindup/sss_ProportionalAction ==
  lb_genFdfw : Inport
  lb_genInpErr : Inport  Port=2
  lb_genInitCond : Inport  Port=3
  lb_genPropGain : Inport  Port=4
  lb_bolRset : Inport  Port=5
  lb_genLowLim : Inport  Port=6
  lb_genUpLim : Inport  Port=7
  Add : Sum  RndMeth=Simplest  OutDataTypeStr=Inherit: Same as first input
  Data Type Duplicate : DataTypeDuplicate
  Data Type Duplicate2 : DataTypeDuplicate  NumInputPorts=3
  Product : Product  OutDataTypeStr=Inherit: Inherit via back propagation  RndMeth=Simplest
  Switch1 : Switch  Criteria=u2 ~= 0  OutDataTypeStr=Inherit: Inherit via back propagation  SaturateOnIntegerOverflow=off  InputSameDT=off
  lib_Conversion_1 : lib_conversion/lib_Conversion_0  lb_parDataType=lb_parOutpDataType  lb_parOutpMaxVal=[]  lb_parOutpMinVal=[]  lb_parSatFlag=off
  lib_DynamicSaturator_0 : lib_dynamic_saturator/lib_DynamicSaturator_0
  lb_satFdfwPlusPropActn : Outport
  wires:
  [lb_bolRset] -> Switch1/2
  [lb_genFdfw] -> Data Type Duplicate/1, Add/1
  lib_DynamicSaturator_0/1 -> lib_Conversion_1/1
  Product/1 -> Data Type Duplicate/2, Add/2  "lb_propActn"
  [lb_genInitCond] -> Switch1/1
  [lb_genInpErr] -> Product/2
  Add/1 -> Switch1/3  "lb_fdfwPlusPropActn"
  lib_Conversion_1/1 -> lb_satFdfwPlusPropActn/1
  Switch1/1 -> lib_DynamicSaturator_0/2, Data Type Duplicate2/1  "lb_unSatFdfwPlusPropActn"
  [lb_genPropGain] -> Product/1
  [lb_genUpLim] -> Data Type Duplicate2/2, lib_DynamicSaturator_0/1
  [lb_genLowLim] -> lib_DynamicSaturator_0/3, Data Type Duplicate2/3
  lb_genInitCond/1 -> [lb_genInitCond]
  lb_genUpLim/1 -> [lb_genUpLim]
  lb_genLowLim/1 -> [lb_genLowLim]
  lb_genFdfw/1 -> [lb_genFdfw]
  lb_genInpErr/1 -> [lb_genInpErr]
  lb_bolRset/1 -> [lb_bolRset]
  lb_genPropGain/1 -> [lb_genPropGain]

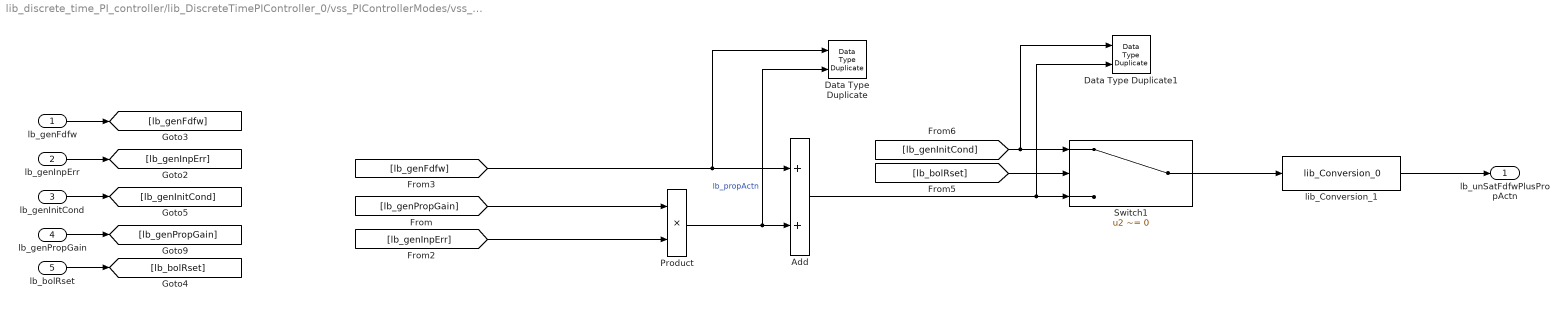
== system lib_discrete_time_PI_controller/lib_DiscreteTimePIController_0/vss_PIControllerModes/vss_SaturationNoAntiWindup/sss_ProportionalAction ==
  lb_genFdfw : Inport
  lb_genInpErr : Inport  Port=2
  lb_genInitCond : Inport  Port=3
  lb_genPropGain : Inport  Port=4
  lb_bolRset : Inport  Port=5
  Add : Sum  RndMeth=Simplest  OutDataTypeStr=Inherit: Same as first input
  Data Type Duplicate : DataTypeDuplicate
  Data Type Duplicate1 : DataTypeDuplicate
  Product : Product  OutDataTypeStr=Inherit: Inherit via back propagation  RndMeth=Simplest
  Switch1 : Switch  Criteria=u2 ~= 0  OutDataTypeStr=Inherit: Inherit via back propagation  SaturateOnIntegerOverflow=off  InputSameDT=off
  lib_Conversion_1 : lib_conversion/lib_Conversion_0  lb_parDataType=lb_parOutpDataType  lb_parOutpMaxVal=[]  lb_parOutpMinVal=[]  lb_parSatFlag=off
  lb_unSatFdfwPlusPropActn : Outport
  wires:
  lb_genInitCond/1 -> [lb_genInitCond]
  Add/1 -> Data Type Duplicate1/2, Switch1/3
  [lb_genInpErr] -> Product/2
  [lb_genFdfw] -> Add/1, Data Type Duplicate/1
  Product/1 -> Add/2, Data Type Duplicate/2  "lb_propActn"
  lb_genFdfw/1 -> [lb_genFdfw]
  lb_genInpErr/1 -> [lb_genInpErr]
  [lb_bolRset] -> Switch1/2
  [lb_genInitCond] -> Data Type Duplicate1/1, Switch1/1
  Switch1/1 -> lib_Conversion_1/1
  lb_bolRset/1 -> [lb_bolRset]
  lib_Conversion_1/1 -> lb_unSatFdfwPlusPropActn/1
  lb_genPropGain/1 -> [lb_genPropGain]
  [lb_genPropGain] -> Product/1
